simulink model "syntheticFlow_th"  (R2022a)
settings: Solver=FixedStepAuto  StartTime=0.0  StopTime=env.water.tFinData.Value  RelTol=1e-3
libraries: syntheticFlow_ul x1
settings Model: Creator=Ayaz  LastModifiedBy=lhill8
settings SolverCC: AlgebraicLoopSolver=TrustRegion
settings DebuggingCC: UnconnectedInputMsg=warning  UnconnectedOutputMsg=warning  UnconnectedLineMsg=warning  SFMachineParentedDataDiag=warning

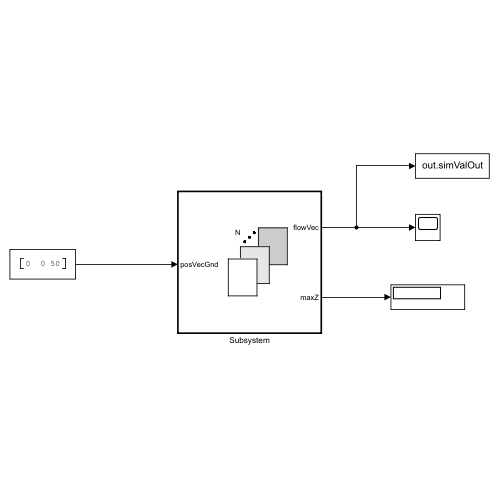
[thumbnail: Simulink's stored preview of the top-level diagram]
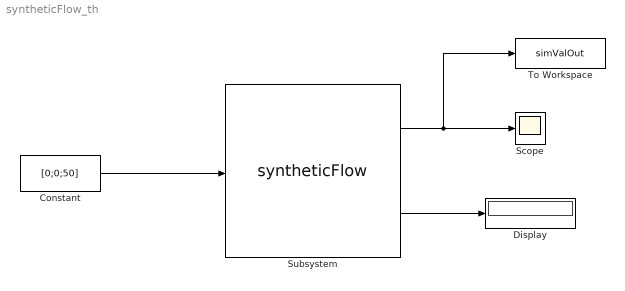
== system syntheticFlow_th ==
  Constant : Constant  Value=[0;0;50]
  Display : Display
  Scope : Scope
  Subsystem : syntheticFlow_ul/syntheticFlow  en=env
  To Workspace : ToWorkspace  VariableName=simValOut  SaveFormat=Timeseries  SampleTime=-1
  wires:
  Constant/1 -> Subsystem/1
  Subsystem/1 -> To Workspace/1, Scope/1
  Subsystem/2 -> Display/1
